simulink model "CurrentLoading_Simulation"  (R2024b)
settings: Solver=FixedStepAuto  StartTime=0.0  StopTime=100  FixedStep=1/(ADC_SamplingRate)  MaxStep=0.01  RelTol=1e-3
values from neighbouring files (symbols this model uses):
  ADC_SamplingRate = 5000    [parameters.m]
undefined symbols (not defined in the file or in its folder): R_sim, VCCS
libraries: fl_lib x12, nesl_utility x4, ee_lib x2
settings Model: STM32="{\"CORDICDriver\":[{\"ID\":\"CurrentLoading_Simulation:658:4:832\"},{\"ID\":\"CurrentLoading_Simulation:658:4:834\"}]}"  Creator=JesseJabezArendse  LastModifiedBy=JesseJabezArendse
settings SolverCC: MaxConsecutiveMinStep=1000  ShapePreserveControl=EnableAll  ZeroCrossControl=EnableAll  ZeroCrossAlgorithm=Adaptive
settings DebuggingCC: MaskedZcDiagnostic=none  IgnoredZcDiagnostic=none
settings RTWCC: GPUComputeCapability=3.5
settings SimscapeCC: ExplicitSolverDiagnosticOptions=none  SimscapeCompileComponentReuse=on

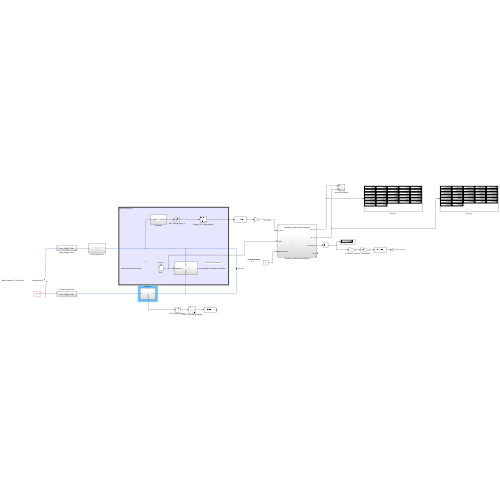
[thumbnail: Simulink's stored preview of the top-level diagram]
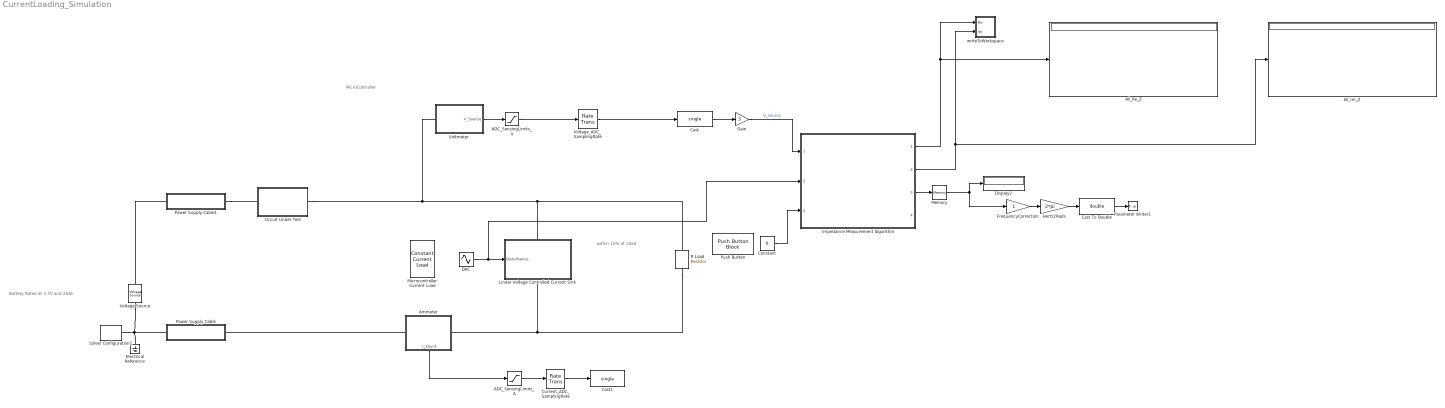
== system CurrentLoading_Simulation ==
  note: within 10% of rated
  note: Battery Rated at 3.7V and 20Ah
  note: MicroController
  ADC_SensingLimits_A : Saturate  UpperLimit=3.3  LowerLimit=-3.3  OutDataTypeStr=Inherit: Inherit via back propagation
  ADC_SensingLimits_V : Saturate  UpperLimit=3.3  LowerLimit=-3.3
  All_Im_Z : Display
  All_Re_Z : Display
  Ammeter : Subsystem
      settings: PortSchema="{\"entries\":[{\"content\":{\"sides\":[{\"content\":{\"connectorIds\":[\"LConn1\"]},\"type\":\"ConnectorPlacement.EquallySpacedRectSide\",\"uuid\":\"34e98bc6-6918-438c-82ce-c7417ebbb64f\"},{\"content\":{\"connectorIds\":[\"RConn1\"],\"side\":\"RIGHT\"},\"type\":\"ConnectorPlacement.EquallySpacedRectSide\",\"uuid\":\"c1762f54-aa85-4248-ab8b-d2cf4b7ac988\"},{\"content\":{\"connectorIds\":[\"Out1\"],\"side\":\"TOP\"},\"type\":\"ConnectorPlacement.EquallySpacedRectSide\",\"uuid\":\"e8622b01-c26e-4f48-80fb-795dda3b9d9b\"}]},\"type\":\"ConnectorPlacement.EquallySpacedConnector\",\"uuid\":\"844fd47f-11fb-4190-ae39-7d566178bd30\"}],\"packageUris\":[\"http://schema.mathworks.com/mf0/Connector/R2020b\"],\"version\":\"1.0\"}"
  Cast : DataTypeConversion  OutDataTypeStr=single  SaturateOnIntegerOverflow=off  RndMeth=Floor
  Cast To Double : DataTypeConversion  OutDataTypeStr=double  SaturateOnIntegerOverflow=off  RndMeth=Floor
  Cast1 : DataTypeConversion  OutDataTypeStr=single  SaturateOnIntegerOverflow=off  RndMeth=Floor
  Circuit Under Test : Subsystem
  Constant : Constant  Value=0  OutDataTypeStr=boolean
  Current_ADC_SamplingRate : RateTransition  Deterministic=off  OutPortSampleTime=1/ADC_SamplingRate
  DAC : Sin  Amplitude=VCCS.Ic/2  Bias=VCCS.Ic/2  Frequency=1.0  Phase=-pi/2  SampleTime=0
  Display2 : Display
  Electrical Reference : fl_lib/Electrical/Electrical Elements/Electrical Reference
  FrequencyCorrection : Gain
  Gain : Gain  Gain=3
  Hertz2Rads : Gain  Gain=2*pi
  Impedance Measurement Algorithm : Subsystem  ReferencedSubsystem=Impedance_Measurement_Algorithm
  Linear Voltage Controlled Current Sink : Subsystem
      settings: PortSchema="{\"entries\":[{\"content\":{\"sides\":[{\"content\":{\"connectorIds\":[\"In1\"]},\"type\":\"ConnectorPlacement.EquallySpacedRectSide\",\"uuid\":\"18d529a9-1cf8-4422-88d7-d8552fbc69b1\"},{\"content\":{\"side\":\"RIGHT\"},\"type\":\"ConnectorPlacement.EquallySpacedRectSide\",\"uuid\":\"d099dce7-fb34-4cde-a1aa-9938a0a6f030\"},{\"content\":{\"connectorIds\":[\"LConn1\"],\"side\":\"TOP\"},\"type\":\"ConnectorPlacement.EquallySpacedRectSide\",\"uuid\":\"f8047e6b-d66f-4a7e-8493-e8033d6b44b9\"},{\"content\":{\"connectorIds\":[\"RConn1\"],\"side\":\"BOTTOM\"},\"type\":\"ConnectorPlacement.EquallySpacedRectSide\",\"uuid\":\"82df79ce-b48a-4c65-8b98-c5c94047aaf0\"}]},\"type\":\"ConnectorPlacement.EquallySpacedConnector\",\"uuid\":\"b1df41be-ee9b-457e-b8ab-8cc4e6bfe837\"}],\"packageUris\":[\"http://schema.mathworks.com/mf0/Connector/R2020b\"],\"version\":\"1.0\"}"
  Memory : Memory
  Microcontroller Current Load : ee_lib/Passive/Constant Current Load  load_type=ee.enum.dc_ac.dc  consumed_current=0.11 A  min_supply_voltage=3.3 V  G_reverse=1e-6 S  deltaV=1e-3 V  consumed_current_rms=100 A  f0=60 Hz  Vrms_min=200 V  fault_action=simscape.enum.assert.action.none  t_fault=1 s
      settings: InternalSimscapePortConfiguration="{\"Bottom\":[],\"Left\":[{\"id\":\"p\",\"label\":\"+\",\"type\":\"foundation.electrical.electrical\"}],\"Right\":[{\"id\":\"n\",\"label\":\"-\",\"type\":\"foundation.electrical.electrical\"}],\"Top\":[]}"
  Parameter Writer1 : ParameterWriter  ParameterOwnerBlock=../DAC  ParameterName=Frequency  ParameterInternalName=Frequency
  Power Supply Cable : Subsystem  ReferencedSubsystem=Power_Supply_Cable
  Power Supply Cable1 : Subsystem  ReferencedSubsystem=Power_Supply_Cable
  Push Button : PushButtonBlock  OffValue=0.000000
  R Load : fl_lib/Electrical/Electrical Elements/Resistor  R=30 Ohm  i_specify=off  i_priority=None  i=0 A  i_nominal_specify=off  i_nominal_value=1  i_nominal_unit=A  v_specify=off  v_priority=None  v=0 V  v_nominal_specify=off  v_nominal_value=1  v_nominal_unit=V
  Solver Configuration1 : nesl_utility/Solver Configuration  PhysicalDomain=network_engine_domain  SubClassName=solver  LeftPortType=input  RightPortType=generic  Tones=[]  Harmonics=[]  SimulateNoise=off  Profile=off  UseLocalSampling=off  EnableSwitchedLinearOptims=on  FrequencyDomain=off  UseCCode=off  RelTol=0.001  AbsTol=0.001  MinStep=1e-09  ToWorkspace=off  RevertToSquareIcSolve=off  NumHomotopyIterations=100  PhasorMode=off  PhasorModeNumHarmonics=1  ConsistencySolver=NEWTON_XTOL_AFTER_FTOL  IndexReductionMethod=None  DoDC=on  ResidualTolerance=1e-09  ConsistencyTolSource=GLOBAL  ConsistencyAbsTol=0.001  ConsistencyRelTol=0.001  ConsistencyTolFactor=0.001  UseLocalSolver=on  LocalSolverChoice=NE_BACKWARD_EULER_ADVANCER  ResolveIndetEquations=off  FunctionEvalNumThread=1  LocalSolverSampleTime=1/ADC_SamplingRate  DoFixedCost=off  MaxNonlinIter=3  MaxModeIter=2  ComputeImpulses=off  ImpulseIterations=2  LinearAlgebra=auto  LinearAlgebraNumThread=0  EquationFormulation=NE_TIME_EF  DelaysMemoryBudget=1024  AutomaticFiltering=off  FilteringTimeConstant=0.001  PartitionStorageMethod=AS_NEEDED  PartitionMemoryBudget=1024  PartitionMethod=ROBUST  MultibodyUseLocalSolver=off  MultibodyLocalSolverChoice=ODE1  MultibodyLocalSolverSampleTime=0.001
  Voltage Source : ee_lib/Sources/Voltage Source  dc_voltage=Batt.OCV V  ac_voltage=0 V  ac_shift=0 rad  ac_frequency=60 Hz  noise_mode=ee.enum.sources.noise.Disabled  PSD=0.000000001 V^2/Hz  sample_time=1e-3 s  repeatability=ee.enum.sources.repeatability.NotRepeatable  user_seed=0  auto_seed=3499211588  i_specify=off  i_priority=None  i=0 A  i_nominal_specify=off  i_nominal_value=1  i_nominal_unit=A  v_specify=off  v_priority=None  v=0 V  v_nominal_specify=off  v_nominal_value=1  v_nominal_unit=V
  Voltage_ADC_SamplingRate : RateTransition  Deterministic=off  OutPortSampleTime=1/ADC_SamplingRate
  Voltmeter : Subsystem
  writeToWorkspace : Subsystem
  wires:
  Impedance Measurement Algorithm/3 -> Memory/1
  Impedance Measurement Algorithm/1 -> All_Re_Z/1, writeToWorkspace/1(Re)
  Hertz2Rads/1 -> Cast To Double/1
  Constant/1 -> Impedance Measurement Algorithm/3
  Memory/1 -> FrequencyCorrection/1, Display2/1
  Impedance Measurement Algorithm/2 -> All_Im_Z/1, writeToWorkspace/2(Im)
  Voltage_ADC_SamplingRate/1 -> Cast/1
  Current_ADC_SamplingRate/1 -> Cast1/1
  FrequencyCorrection/1 -> Hertz2Rads/1
  DAC/1 -> Impedance Measurement Algorithm/2, Linear Voltage Controlled Current Sink/1(Disturbance)
  Voltmeter/1(V_Source) -> ADC_SensingLimits_V/1
  Ammeter/1(I_Shunt) -> ADC_SensingLimits_A/1
  ADC_SensingLimits_V/1 -> Voltage_ADC_SamplingRate/1
  ADC_SensingLimits_A/1 -> Current_ADC_SamplingRate/1
  Cast To Double/1 -> Parameter Writer1/1
  Gain/1 -> Impedance Measurement Algorithm/1  "V_source"
  Cast/1 -> Gain/1
  connections:
  R Load/RConn1 -- Linear Voltage Controlled Current Sink/RConn1 -- Ammeter/LConn1
  Power Supply Cable1/LConn1 -- Voltage Source/LConn1
  Voltmeter/LConn1 -- Circuit Under Test/RConn1 -- R Load/LConn1 -- Linear Voltage Controlled Current Sink/LConn1
  Power Supply Cable/RConn1 -- Voltage Source/RConn1 -- Electrical Reference/LConn1 -- Solver Configuration1/RConn1
  Ammeter/RConn1 -- Power Supply Cable/LConn1
  Power Supply Cable1/RConn1 -- Circuit Under Test/LConn1

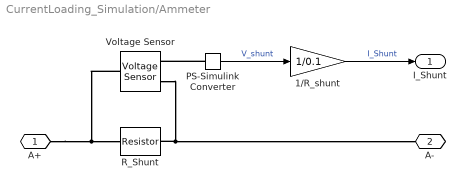
== system CurrentLoading_Simulation/Ammeter ==
  1/R_shunt : Gain  Gain=1/0.1
  PS-Simulink Converter : nesl_utility/PS-Simulink Converter  PhysicalDomain=network_engine_domain  SubClassName=ps_output  LeftPortType=input  RightPortType=output  PseudoPeriodic=off  Frequencies=[]  VectorFormat=inherit  Unit=inherit  AffineConversion=off
  R_Shunt : fl_lib/Electrical/Electrical Elements/Resistor  R=0.1 Ohm  i_specify=off  i_priority=None  i=0 A  i_nominal_specify=off  i_nominal_value=1  i_nominal_unit=A  v_specify=off  v_priority=None  v=0 V  v_nominal_specify=off  v_nominal_value=1  v_nominal_unit=V
  Voltage Sensor : fl_lib/Electrical/Electrical Sensors/Voltage Sensor
  A+ : PMIOPort  Side=Left
  A- : PMIOPort  Port=2  Side=Right
  I_Shunt : Outport
  wires:
  PS-Simulink Converter/1 -> 1/R_shunt/1  "V_shunt"
  1/R_shunt/1 -> I_Shunt/1  "I_Shunt"
  connections:
  Voltage Sensor/LConn1 -- A+/RConn1 -- R_Shunt/LConn1
  PS-Simulink Converter/LConn1 -- Voltage Sensor/RConn1
  Voltage Sensor/RConn2 -- A-/RConn1 -- R_Shunt/RConn1

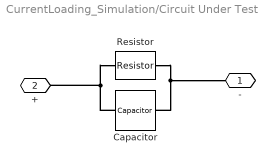
== system CurrentLoading_Simulation/Circuit Under Test ==
  Capacitor : fl_lib/Electrical/Electrical Elements/Capacitor  c=C_sim F  r=1e-6 Ohm  g=0 1/Ohm  i_specify=off  i_priority=None  i=0 A  i_nominal_specify=off  i_nominal_value=1  i_nominal_unit=A  v_specify=off  v_priority=None  v=0 V  v_nominal_specify=off  v_nominal_value=1  v_nominal_unit=V  vc_specify=off  vc_priority=High  vc=0 V  vc_nominal_specify=off  vc_nominal_value=1  vc_nominal_unit=V
  Resistor : fl_lib/Electrical/Electrical Elements/Resistor  R=R_sim Ohm  i_specify=off  i_priority=None  i=0 A  i_nominal_specify=off  i_nominal_value=1  i_nominal_unit=A  v_specify=off  v_priority=None  v=0 V  v_nominal_specify=off  v_nominal_value=1  v_nominal_unit=V
  - : PMIOPort  Side=Right
  + : PMIOPort  Port=2  Side=Left
  connections:
  Capacitor/LConn1 -- +/RConn1 -- Resistor/LConn1
  Resistor/RConn1 -- Capacitor/RConn1 -- -/RConn1

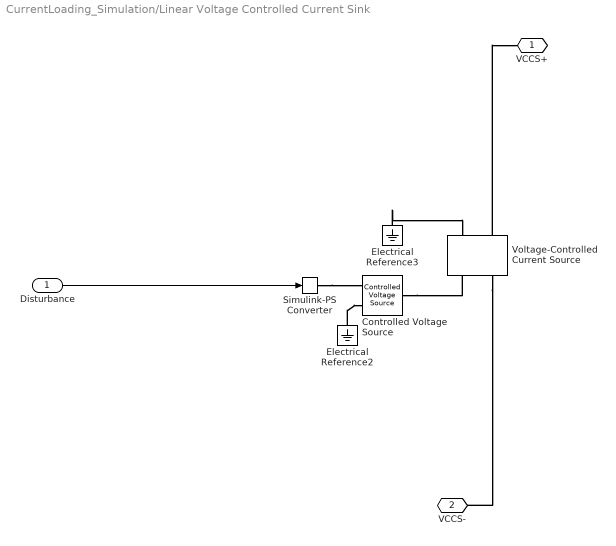
== system CurrentLoading_Simulation/Linear Voltage Controlled Current Sink ==
  Disturbance : Inport
  Controlled Voltage Source : fl_lib/Electrical/Electrical Sources/Controlled Voltage Source
  Electrical Reference2 : fl_lib/Electrical/Electrical Elements/Electrical Reference
  Electrical Reference3 : fl_lib/Electrical/Electrical Elements/Electrical Reference
  Simulink-PS Converter : nesl_utility/Simulink-PS Converter  PhysicalDomain=network_engine_domain  SubClassName=ps_input  LeftPortType=input  RightPortType=output  PseudoPeriodic=off  Frequencies=[]  NoiseDistribution=none  NoiseParameters=[]  Unit=1  AffineConversion=off  FilteringAndDerivatives=provide  SimscapeFilterOrder=1  InputFilterTimeConstant=0.001  UdotUserProvided=0
  Voltage-Controlled Current Source : fl_lib/Electrical/Electrical Sources/Voltage-Controlled Current Source  K=1 1/Ohm  v1_specify=off  v1_priority=None  v1=0 V  v1_nominal_specify=off  v1_nominal_value=1  v1_nominal_unit=V  i2_specify=off  i2_priority=None  i2=0 A  i2_nominal_specify=off  i2_nominal_value=1  i2_nominal_unit=A
      settings: InternalSimscapePortConfiguration="{\"Bottom\":[],\"Left\":[{\"id\":\"p1\",\"label\":\"+\",\"type\":\"foundation.electrical.electrical\"},{\"id\":\"head\",\"label\":\"\",\"type\":\"foundation.electrical.electrical\"}],\"Right\":[{\"id\":\"n1\",\"label\":\"-\",\"type\":\"foundation.electrical.electrical\"},{\"id\":\"tail\",\"label\":\"\",\"type\":\"foundation.electrical.electrical\"}],\"Top\":[]}"
  VCCS+ : PMIOPort  Side=Left
  VCCS- : PMIOPort  Port=2  Side=Right
  wires:
  Disturbance/1 -> Simulink-PS Converter/1
  connections:
  Controlled Voltage Source/LConn1 -- Voltage-Controlled Current Source/LConn1
  Electrical Reference3/LConn1 -- Voltage-Controlled Current Source/RConn1
  Simulink-PS Converter/RConn1 -- Controlled Voltage Source/RConn1
  Voltage-Controlled Current Source/LConn2 -- VCCS-/RConn1
  Voltage-Controlled Current Source/RConn2 -- VCCS+/RConn1
  Electrical Reference2/LConn1 -- Controlled Voltage Source/RConn2

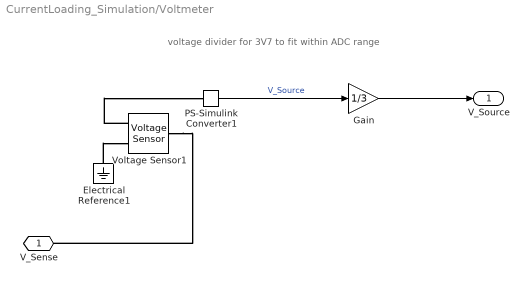
== system CurrentLoading_Simulation/Voltmeter ==
  note: voltage divider for 3V7 to fit within ADC range
  Electrical Reference1 : fl_lib/Electrical/Electrical Elements/Electrical Reference
  Gain : Gain  Gain=1/3
  PS-Simulink Converter1 : nesl_utility/PS-Simulink Converter  PhysicalDomain=network_engine_domain  SubClassName=ps_output  LeftPortType=input  RightPortType=output  PseudoPeriodic=off  Frequencies=[]  VectorFormat=inherit  Unit=inherit  AffineConversion=off
  Voltage Sensor1 : fl_lib/Electrical/Electrical Sensors/Voltage Sensor
  V_Sense : PMIOPort  Side=Left
  V_Source : Outport
  wires:
  PS-Simulink Converter1/1 -> Gain/1  "V_Source"
  Gain/1 -> V_Source/1
  connections:
  Electrical Reference1/LConn1 -- Voltage Sensor1/RConn2
  Voltage Sensor1/RConn1 -- PS-Simulink Converter1/LConn1
  Voltage Sensor1/LConn1 -- V_Sense/RConn1

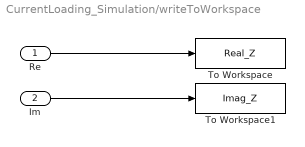
== system CurrentLoading_Simulation/writeToWorkspace ==
  Re : Inport
  Im : Inport  Port=2
  To Workspace : ToWorkspace  VariableName=Real_Z  SampleTime=-1
  To Workspace1 : ToWorkspace  VariableName=Imag_Z  SampleTime=-1
  wires:
  Im/1 -> To Workspace1/1
  Re/1 -> To Workspace/1
